simulink model "X_Model"  (R2017a)
settings: Solver=VariableStepAuto  StartTime=0.0  StopTime=sim_time  RelTol=1e-3
values from neighbouring files (symbols this model uses):
  D_Model_SISO = cell(6,1)    [DigitalControlsProject1.m]
  IC = [0.02; 0.03]    [DigitalControlsProject1.m]
  K_test = cell(6,1)    [DigitalControlsProject1.m]
  N = cell(6,1)    [DigitalControlsProject1.m]
  T = 1/40    (= 0.025)    [DigitalControlsProject1.m]
settings Model: Creator=Alphakyl  LastModifiedBy=windo

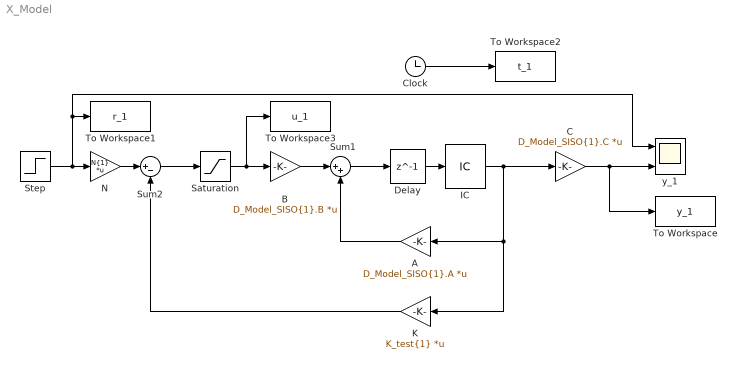
== system X_Model ==
  A : Gain  Gain=D_Model_SISO{1}.A  Multiplication=Matrix(K*u)
  B : Gain  Gain=D_Model_SISO{1}.B  Multiplication=Matrix(K*u)
  C : Gain  Gain=D_Model_SISO{1}.C  Multiplication=Matrix(K*u)
  Clock : Clock
  Delay : Delay  DelayLength=1  SampleTime=T
  IC : InitialCondition  Value=IC
  K : Gain  Gain=K_test{1}  Multiplication=Matrix(K*u)
  N : Gain  Gain=N{1}  Multiplication=Matrix(K*u)
  Saturation : Saturate  UpperLimit=100  LowerLimit=-100
  Step : Step  SampleTime=T
  Sum1 : Sum  Inputs=|++
  Sum2 : Sum  Inputs=|+-
  To Workspace : ToWorkspace  VariableName=y_1  SampleTime=-1
  To Workspace1 : ToWorkspace  VariableName=r_1  SampleTime=-1
  To Workspace2 : ToWorkspace  VariableName=t_1  SampleTime=-1
  To Workspace3 : ToWorkspace  VariableName=u_1  SampleTime=-1
  "y_1 " : Scope  NumInputPorts=2
  wires:
  Delay/1 -> IC/1
  A/1 -> Sum1/2
  B/1 -> Sum1/1
  Sum2/1 -> Saturation/1
  K/1 -> Sum2/2
  Step/1 -> To Workspace1/1, "y_1 "/1, N/1
  C/1 -> To Workspace/1, "y_1 "/2
  N/1 -> Sum2/1
  Clock/1 -> To Workspace2/1
  Saturation/1 -> To Workspace3/1, B/1
  Sum1/1 -> Delay/1
  IC/1 -> A/1, K/1, C/1
